simulink model "CCpath"  (R2016b)
settings: Solver=VariableStepAuto  StartTime=0.0  StopTime=10.0  RelTol=1e-3
settings Model: Creator=karanverma  LastModifiedBy=karanverma

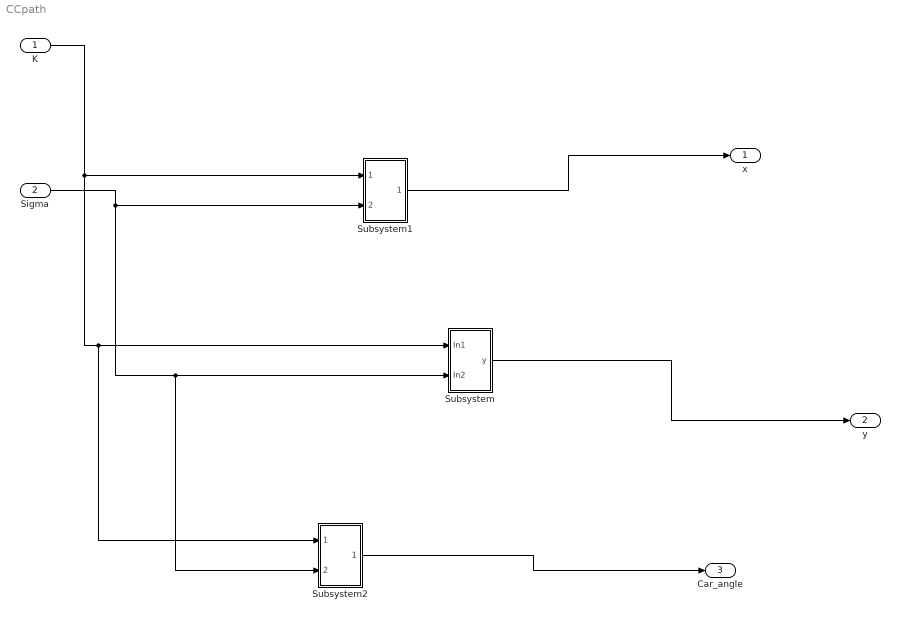
== system CCpath ==
  K : Inport
  Sigma : Inport  Port=2
  Subsystem : Subsystem
  Subsystem1 : Subsystem
  Subsystem2 : Subsystem
  x : Outport
  y : Outport  Port=2
  Car_angle : Outport  Port=3
  wires:
  K/1 -> Subsystem1/1(In1), Subsystem2/1(In1), Subsystem/1(In1)
  Sigma/1 -> Subsystem1/2(In2), Subsystem2/2(In2), Subsystem/2(In2)
  Subsystem/1(y) -> y/1
  Subsystem1/1(Out1) -> x/1
  Subsystem2/1(Out1) -> Car_angle/1

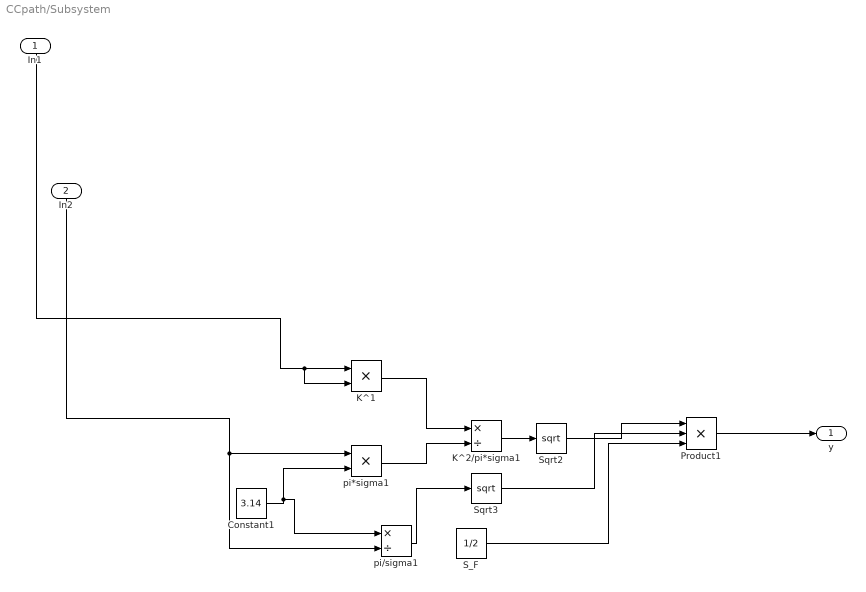
== system CCpath/Subsystem ==
  In1 : Inport
  In2 : Inport  Port=2
  Constant1 : Constant  Value=3.14
  K^1 : Product
  K^2/pi*sigma1 : Product  Inputs=*/
  Product1 : Product  Inputs=3
  S_F : Constant  Value=1/2
  Sqrt2 : Sqrt  SaturateOnIntegerOverflow=on
  Sqrt3 : Sqrt  SaturateOnIntegerOverflow=on
  pi*sigma1 : Product
  pi/sigma1 : Product  Inputs=*/
  y : Outport
  wires:
  Constant1/1 -> pi/sigma1/1, pi*sigma1/2
  K^1/1 -> K^2/pi*sigma1/1
  pi*sigma1/1 -> K^2/pi*sigma1/2
  K^2/pi*sigma1/1 -> Sqrt2/1
  Sqrt2/1 -> Product1/1
  pi/sigma1/1 -> Sqrt3/1
  S_F/1 -> Product1/3
  Sqrt3/1 -> Product1/2
  Product1/1 -> y/1
  In2/1 -> pi/sigma1/2, pi*sigma1/1
  In1/1 -> K^1/2, K^1/1

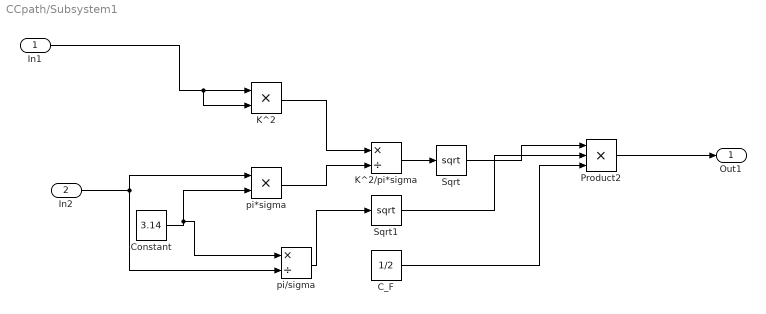
== system CCpath/Subsystem1 ==
  In1 : Inport
  In2 : Inport  Port=2
  C_F : Constant  Value=1/2
  Constant : Constant  Value=3.14
  K^2 : Product
  K^2/pi*sigma : Product  Inputs=*/
  Product2 : Product  Inputs=3
  Sqrt : Sqrt  SaturateOnIntegerOverflow=on
  Sqrt1 : Sqrt  SaturateOnIntegerOverflow=on
  pi*sigma : Product
  pi/sigma : Product  Inputs=*/
  Out1 : Outport
  wires:
  Sqrt1/1 -> Product2/2
  pi*sigma/1 -> K^2/pi*sigma/2
  Product2/1 -> Out1/1
  Constant/1 -> pi/sigma/1, pi*sigma/2
  In2/1 -> pi*sigma/1, pi/sigma/2
  In1/1 -> K^2/2, K^2/1
  K^2/1 -> K^2/pi*sigma/1
  Sqrt/1 -> Product2/1
  pi/sigma/1 -> Sqrt1/1
  C_F/1 -> Product2/3
  K^2/pi*sigma/1 -> Sqrt/1

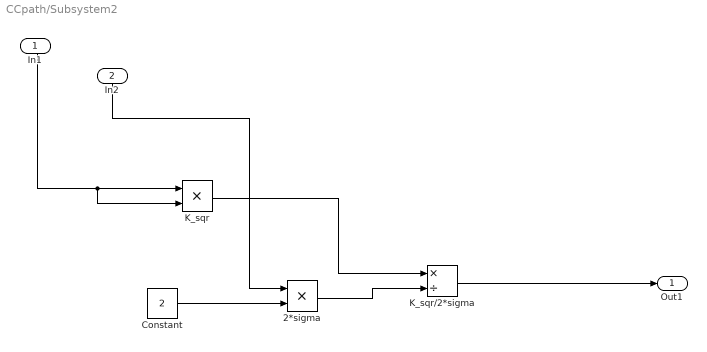
== system CCpath/Subsystem2 ==
  In1 : Inport
  In2 : Inport  Port=2
  2*sigma : Product
  Constant : Constant  Value=2
  K_sqr : Product
  K_sqr/2*sigma : Product  Inputs=*/
  Out1 : Outport
  wires:
  In2/1 -> 2*sigma/1
  In1/1 -> K_sqr/2, K_sqr/1
  Constant/1 -> 2*sigma/2
  K_sqr/2*sigma/1 -> Out1/1
  2*sigma/1 -> K_sqr/2*sigma/2
  K_sqr/1 -> K_sqr/2*sigma/1
